simulink model "sensor_block"  (Simulink 7.4)
settings: Solver=FixedStepDiscrete  StartTime=0  StopTime=inf  FixedStep=0.05  RelTol=1e-3
StartFcn:
  | localAddEventListener
settings Model: Creator=kthwsnt  LastModifiedBy=aitorhh
settings SolverCC: PositivePriorityOrder=on
settings OptimizationCC: InitFltsAndDblsToZero=on
settings SimEventsCC: propDiagAttribOutput=1  propDiagFcnCallOutput=1  propDiagStatOutput=0

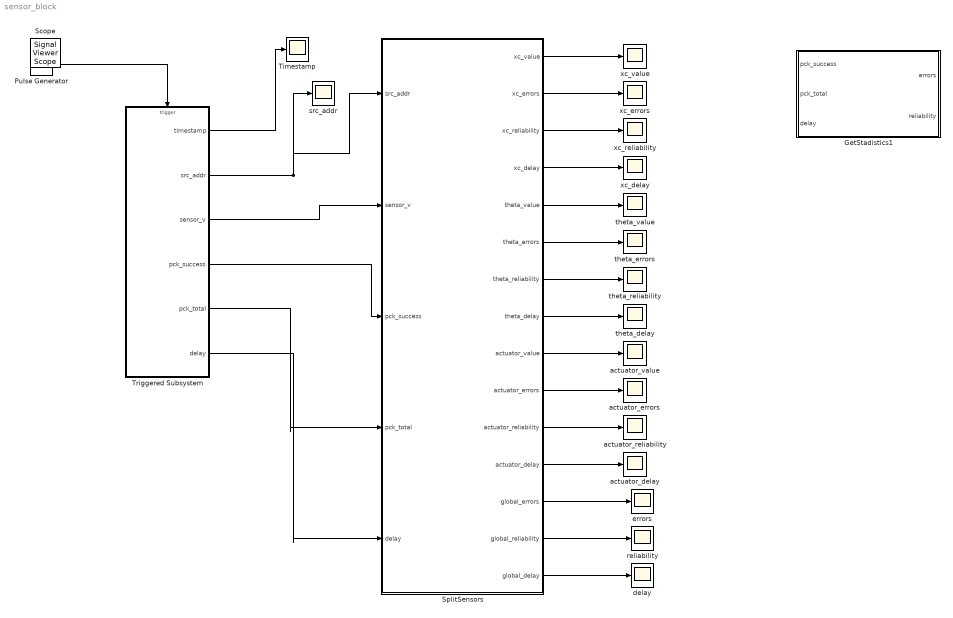
== system sensor_block ==
  GetStadistics1 : Stateflow chart
  Pulse Generator : DiscretePulseGenerator  PulseType=Time based  Amplitude=1  Period=1  PulseWidth=5  PhaseDelay=0  SampleTime=1
  SplitSensors : Stateflow chart
  Timestamp : Scope
      settings: TimeRange=1000  YMin=9.6605e+06  YMax=9.669e+06  SaveName=ScopeData5
  Triggered Subsystem : Subsystem  TreatAsAtomicUnit=on
  actuator_delay : Scope
      settings: TimeRange=1000  YMin=0  YMax=100  SaveName=ScopeData13
  actuator_errors : Scope
      settings: TimeRange=1000  YMin=0  YMax=1  SaveName=ScopeData14
  actuator_reliability : Scope
      settings: TimeRange=1000  YMin=0  YMax=100  SaveName=ScopeData15
  actuator_value : Scope
      settings: TimeRange=1000  YMin=-1  YMax=1  SaveName=ScopeData16
  delay : Scope
      settings: TimeRange=10000  YMin=-1  YMax=1
  errors : Scope
      settings: TimeRange=10000  YMin=-1  YMax=1  SaveName=ScopeData3
  reliability : Scope
      settings: TimeRange=1000  YMin=0.95  YMax=1.05  SaveName=ScopeData2
  src_addr : Scope
      settings: TimeRange=10000  YMin=1  YMax=2
  theta_delay : Scope
      settings: TimeRange=1000  YMin=0  YMax=100  SaveName=ScopeData12
  theta_errors : Scope
      settings: TimeRange=1000  YMin=0  YMax=1  SaveName=ScopeData10
  theta_reliability : Scope
      settings: TimeRange=1000  YMin=0  YMax=100  SaveName=ScopeData11
  theta_value : Scope
      settings: TimeRange=1000  YMin=0  YMax=450  SaveName=ScopeData9
  xc_delay : Scope
      settings: TimeRange=1000  YMin=0  YMax=100  SaveName=ScopeData8
  xc_errors : Scope
      settings: TimeRange=1000  YMin=0  YMax=1  SaveName=ScopeData6
  xc_reliability : Scope
      settings: TimeRange=1000  YMin=0  YMax=3  SaveName=ScopeData7
  xc_value : Scope
      settings: TimeRange=1000  YMin=6.02922  YMax=6.02922  SaveName=ScopeData4
  Scope : SignalViewerScope  IOType=viewer  RefreshTime=0.035000
      settings: YMin=4660  YMax=4660
  wires:
  Pulse Generator/1 -> Triggered Subsystem/Trigger
  Triggered Subsystem/2(src_addr) -> src_addr/1, SplitSensors/1(src_addr)
  Triggered Subsystem/3(sensor_v) -> SplitSensors/2(sensor_v)
  Triggered Subsystem/1(timestamp) -> Timestamp/1
  Triggered Subsystem/6(delay) -> SplitSensors/5(delay)
  SplitSensors/14(global_reliability) -> reliability/1
  SplitSensors/13(global_errors) -> errors/1
  SplitSensors/15(global_delay) -> delay/1
  Triggered Subsystem/5(pck_total) -> SplitSensors/4(pck_total)
  Triggered Subsystem/4(pck_success) -> SplitSensors/3(pck_success)
  SplitSensors/1(xc_value) -> xc_value/1
  SplitSensors/7(theta_reliability) -> theta_reliability/1
  SplitSensors/6(theta_errors) -> theta_errors/1
  SplitSensors/5(theta_value) -> theta_value/1
  SplitSensors/4(xc_delay) -> xc_delay/1
  SplitSensors/2(xc_errors) -> xc_errors/1
  SplitSensors/3(xc_reliability) -> xc_reliability/1
  SplitSensors/8(theta_delay) -> theta_delay/1
  SplitSensors/12(actuator_delay) -> actuator_delay/1
  SplitSensors/11(actuator_reliability) -> actuator_reliability/1
  SplitSensors/10(actuator_errors) -> actuator_errors/1
  SplitSensors/9(actuator_value) -> actuator_value/1

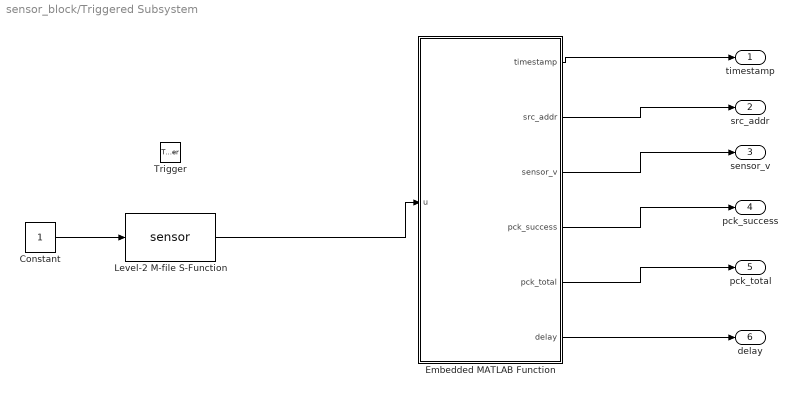
== system sensor_block/Triggered Subsystem ==
  Trigger : TriggerPort
  Constant : Constant  OutDataType=fixdt(1, 16)  OutScaling=2^0
  Embedded MATLAB Function : Stateflow chart
  Level-2 M-file S-Function : M-S-Function  FunctionName=sensor
  timestamp : Outport  OutDataType=sfix(16)  OutScaling=2^0
  src_addr : Outport  Port=2  OutDataType=sfix(16)  OutScaling=2^0
  sensor_v : Outport  Port=3  OutDataType=sfix(16)  OutScaling=2^0
  pck_success : Outport  Port=4  OutDataType=sfix(16)  OutScaling=2^0
  pck_total : Outport  Port=5  OutDataType=sfix(16)  OutScaling=2^0
  delay : Outport  Port=6  OutDataType=sfix(16)  OutScaling=2^0
  wires:
  Constant/1 -> Level-2 M-file S-Function/1
  Level-2 M-file S-Function/1 -> Embedded MATLAB Function/1(u)
  Embedded MATLAB Function/1(timestamp) -> timestamp/1
  Embedded MATLAB Function/2(src_addr) -> src_addr/1
  Embedded MATLAB Function/3(sensor_v) -> sensor_v/1
  Embedded MATLAB Function/4(pck_success) -> pck_success/1
  Embedded MATLAB Function/5(pck_total) -> pck_total/1
  Embedded MATLAB Function/6(delay) -> delay/1

== matlab function Triggered Subsystem/Embedded MATLAB Function ==
  data: u input double; timestamp output double; src_addr output double; sensor_v output double; pck_success output double; pck_total output double; delay output double
function [timestamp, src_addr, sensor_v, pck_success, pck_total, delay] = parsePacket(u)

XCART_ADDRESS = 1;
TPENDULUM_ADDRESS = 2;
% 02    0f     61 88   e7     34 12     03 00      00 00    00 13    04 e3    0f ff    69    c9     00        c0  2d  40  58 
% 02    0f     61 88   d2     34 12     03 00      00 00    00 00    00 00    07 ff    69    c2     84        32 8d de 02 
% 02    0f     61 88   be     34 12     03 00      00 00    00 00    00 00    07 ff    67    ca     00        c4 f0 8d 03 

% id| length|        |seqnum|  PANID  | Src adr | Dst addr | xc    | theta  |  u_out  | lqi | rssi| mhrLen | timestamp
%           
%#eml
% 02   0f     61 88    9f     34 12     00 00      02 00     00 00    00 4b      00 4b      02 04      6b    c2     00       ba 15 28 00 
% id| length|        |seqnum|  PANID  | Dest adr | Src addr | xc    | success |  total  | delay | lqi | rssi| mhrLen | timestamp

l=length(u);
%
% packet information
%
seq_num = u(5);
pan_id = bitor(bitshift(uint16(u(7)),8), uint16(u(6)));
dst_addr = bitor(bitshift(uint16(u(9)),8), uint16(u(8)));
src_addr= bitor(bitshift(uint16(u(11)),8), uint16(u(10)));


%
% Sensors and control voltage
%
% xc_sensor=bitor(bitshift(uint16(u(14)),8), uint16(u(15)))*9.2E-5;
% theta_sensor=bitor(bitshift(uint16(u(12)),8), uint16(u(13))) / 1024.0 * 2 * 3.14159265;
% u_control = bitor(bitshift(uint16(u(16)),8), uint16(u(17)));
% u_control = (u_control / 1638) * 4.8 -6;

% Sensor values
sensor_v = bitor(bitshift(uint16(u(12)),8), uint16(u(13)));
pck_total = bitor(bitshift(uint16(u(14)),8), uint16(u(15)));
pck_success = bitor(bitshift(uint16(u(16)),8), uint16(u(17)));

%pck_total = uint8(u(14));
%pck_success = uint8(u(15));
delay = bitor(bitshift(uint16(u(18)),8), uint16(u(19)));

%
% Timestamps and more packet information
%
lqi=uint16(u(l-6));
rssi=uint16(u(l-5));

timestamp1 = bitor(bitshift(uint32(u(l-1)),24), bitshift(uint32(u(l-2)),16) );
timestamp2 = bitor(bitshift(uint32(u(l-3)),8), uint32(u(l-4) ));
timestamp = bitor(timestamp1, timestamp2)*16E-3; %%in ms

== matlab function SplitSensors ==
  data: src_addr input double; xc_value output double; sensor_v input double; pck_success input double; pck_total input double; delay input double; xc_errors output double; xc_reliability output double; xc_delay output double; theta_value output double; theta_errors output double; theta_reliability output double; theta_delay output double; actuator_value output double; actuator_errors output double; actuator_reliability output double; actuator_delay output double; global_errors output double; global_reliability output double; global_delay output double
function [xc_value, xc_errors, xc_reliability, xc_delay, ...
        theta_value, theta_errors, theta_reliability, theta_delay,...
        actuator_value, actuator_errors, actuator_reliability, actuator_delay,...
        global_errors, global_reliability, global_delay] = ...
        splitSensors(src_addr, sensor_v, pck_success,  pck_total ,delay)
%#eml
% 
persistent xc_value_p  xc_errors_p xc_reliability_p xc_delay_p ...
     theta_value_p theta_errors_p theta_reliability_p theta_delay_p ...
     actuator_value_p actuator_errors_p actuator_reliability_p actuator_delay_p ...
     global_reliability_p;
 
persistent errors_prev errors_window item;
 
COORDINATOR_ADDRESS = 0;
XCART_ADDRESS = 1;
TPENDULUM_ADDRESS = 2;
SLIDING_WINDOW = 100;

TIME_SYMBOL = 1/(2*32678)*1E3;

NUMBER_LINKS = 2;
NUMBER_SENSORS = 2;

% First initialization of the variables
if isempty(xc_value_p)
    
    xc_value_p = double(0);
    xc_reliability_p = double(0);
    xc_delay_p = double(0);
    
    theta_value_p = double(0);
    theta_reliability_p = double(0);
    theta_delay_p = double(0);
    
    actuator_value_p = double(0);
    actuator_reliability_p = double(0);
    actuator_delay_p = double(0);
    
    global_reliability_p = double(1);
    
    errors_window = zeros(NUMBER_SENSORS + NUMBER_LINKS - 1 , 1);
    item = 1;
    errors_prev = zeros(1, NUMBER_SENSORS + NUMBER_LINKS - 1);

end
    xc_errors_p = uint8(0);
    theta_errors_p = uint8(0);  
    actuator_errors_p = uint8(0);  

    
    if ( src_addr <= (NUMBER_SENSORS + NUMBER_LINKS - 1) &&  src_addr > 0 )
        %
        % SENSOR ---- > COORDINATOR
        %
        
        % Set the new values for the desired sensors
        if src_addr == XCART_ADDRESS
            
            if errors_prev(src_addr + 1 ) < (pck_total - pck_success)
                xc_errors_p = uint8(1);
                errors_window(src_addr + 1) = errors_window(src_addr + 1) + 1;
            end
            
            xc_value_p = double(sensor_v);
            %xc_reliability_p = pck_total - pck_success;
            xc_delay_p = double(delay);
            
        elseif src_addr == TPENDULUM_ADDRESS
            
            if errors_prev(src_addr + 1) < (pck_total - pck_success)
                theta_errors_p = uint8(1);
                errors_window(src_addr + 1) = errors_window(src_addr + 1) + 1;
            end
            
            theta_value_p = double(sensor_v);
            
            %theta_reliability_p = pck_success;
            theta_delay_p = double(delay);
            
        elseif src_addr == COORDINATOR_ADDRESS
            %
            % COORDIANTOR ---- > ACTUATOR
            %
            
            if errors_prev(src_addr + 1) < (pck_total - pck_success)
                actuator_errors_p = uint8(1);
                errors_window(src_addr + 1) = errors_window(src_addr + 1) + 1;
            end
            
            actuator_value_p = double(sensor_v);
            
            %theta_reliability_p = pck_success;
            actuator_delay_p = double(delay);
            
        end
        
        errors_prev(src_addr + 1) = pck_total - pck_success;
        
        % Realiability computation
        
        item = item +1;
        if item == SLIDING_WINDOW
            % Update reliability
            global_reliability_p = 1- sum(errors_window)/SLIDING_WINDOW;
            xc_reliability_p = 1- errors_window(1)/SLIDING_WINDOW;
            theta_reliability_p = 1- errors_window(2)/SLIDING_WINDOW;
            
            errors_window(1) = 0;
            errors_window(2) = 0;
            item = 1;
        end
    end

xc_value = xc_value_p * 9.2E-5;
xc_errors = xc_errors_p;
xc_reliability = xc_reliability_p;
xc_delay = xc_delay_p * TIME_SYMBOL;

theta_value = (theta_value_p / 1024.0) * 2 * 3.14159265;
theta_errors = theta_errors_p;
theta_reliability = theta_reliability_p;
theta_delay = theta_delay_p  * TIME_SYMBOL;

actuator_value = actuator_value_p;
actuator_errors = actuator_errors_p;
actuator_reliability = actuator_reliability_p;
actuator_delay = actuator_delay_p * TIME_SYMBOL; 

global_errors = xc_errors_p + theta_errors_p;
global_reliability = global_reliability_p;

global_delay = (xc_delay_p + theta_delay_p + actuator_delay_p)/2;

if global_delay > 100
   global_delay = double(0); 
end
%global_delay = delay;

== matlab function GetStadistics1 ==
  data: pck_success input double; pck_total input double; delay input double; errors output double; reliability output double
function [errors, reliability ] = ...
    getStadistics (pck_success,  pck_total ,delay)
%#eml
% 
persistent errors_window item pckTotalTrack prevTotalPackets;
 
SLIDING_WINDOW = 100;

% First initialization of the variables
if isempty(item)
    errors_window = zeros(SLIDING_WINDOW, 1);
    pckTotalTrack = zeros(SLIDING_WINDOW, 1);
    item = 1;
end

currentItem = mod(item + 1, SLIDING_WINDOW);
% It could be that the number of received packets
% is not the total packets sent, so we need
% to keep track of it.
if (pck_total == 0 || isempty(prevTotalPackets))
    pckTotalTrack(currentItem) = 1;
    prevTotalPackets = pck_total;
else
    pckTotalTrack(currentItem) = pck_total - prevTotalPackets;
end

% if the previous errors in less than the actual value
% it means that we get a need error
if errors_window(item) < (pck_total - pck_success)
    errors_window(currentItem) = (pck_total - pck_success) - errors_window(item);
else
    errors_window(currentItem) = 0;
end

item = currentItem;

%
% Map the outputs
%
errors = errors_window(item);
reliability = 1-sum(errors_window)/(sum(pckTotalTrack));
